simulink model "modelo"  (R2020b)
settings: Solver=ode45  StartTime=0.0  StopTime=10  MaxStep=0.005  RelTol=0.5e-3  EnableMultiTasking=on
undefined symbols (not defined in the file): B, Jt, Ke, Kt, L, Ra
settings Model: Creator=Administrador  LastModifiedBy=andre
settings DataIOCC: LimitDataPoints=on  SaveFormat=Array  SignalLoggingSaveFormat=ModelDataLogs  ReturnWorkspaceOutputs=off
settings OptimizationCC: ExpressionDepthLimit=2147483647  InitFltsAndDblsToZero=on  LifeSpan=inf
settings DebuggingCC: UnderspecifiedInitializationDetection=Classic  MergeDetectMultiDrivingBlocksExec=none  SolverPrmCheckMsg=warning  FcnCallInpInsideContextMsg=warning  StateNameClashWarn=warning  SFUnexpectedBacktrackingDiag=warning  SFNoUnconditionalDefaultTransitionDiag=warning  SFExecutionAtInitializationDiag=none  ArithmeticOperatorsInVariantConditions=warning
settings HardwareCC: ProdBitPerPointer=32  ProdBitPerSizeT=32  ProdBitPerPtrDiffT=32  ProdLargestAtomicFloat=None  ProdIntDivRoundTo=Undefined  ProdEndianess=Unspecified  ProdWordSize=32  ProdHWDeviceType=32-bit Generic
settings ModelReferenceCC: PropagateSignalLabelsOutOfModel=off
settings SFSimCC: SimUseLocalCustomCode=off  CustomCodeUndefinedFunction=UseInterfaceOnly
settings RTWCC: RTWUseLocalCustomCode=off
settings CodeAppCC: StateflowObjectComments=on
settings GRTTargetCC: TargetLangStandard=C89/C90 (ANSI)  CombineOutputUpdateFcns=off  GRTInterface=on
settings ConfigComp: CovMetricSettings=dw  CovSaveCumulativeToWorkspaceVar=on  CovSaveSingleToWorkspaceVar=on  CovExternalEMLEnable=off

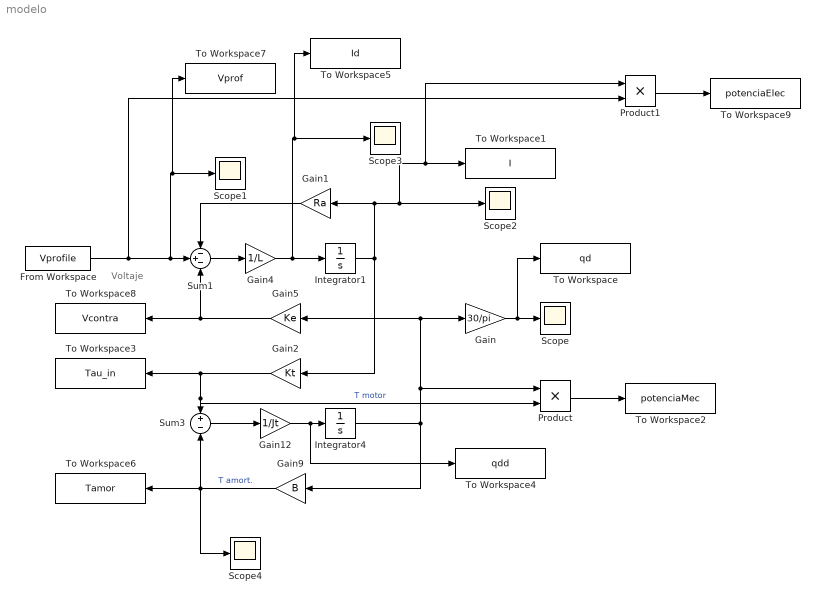
== system modelo ==
  note: Voltaje
  From Workspace : FromWorkspace  VariableName=Vprofile
  Gain : Gain  Gain=30/pi
  Gain1 : Gain  Gain=Ra
  Gain12 : Gain  Gain=1/Jt
  Gain2 : Gain  Gain=Kt
  Gain4 : Gain  Gain=1/L
  Gain5 : Gain  Gain=Ke
  Gain9 : Gain  Gain=B
  Integrator1 : Integrator
  Integrator4 : Integrator
  Product : Product
  Product1 : Product
  Scope{,1..4} (5 alike) : Scope
  Sum1 : Sum  Inputs=-+-
  Sum3 : Sum  Inputs=+-
  To Workspace : ToWorkspace  VariableName=qd  SaveFormat=Timeseries  SampleTime=-1
  To Workspace1 : ToWorkspace  VariableName=I  SaveFormat=Timeseries  SampleTime=-1
  To Workspace2 : ToWorkspace  VariableName=potenciaMec  SaveFormat=Timeseries  SampleTime=-1
  To Workspace3 : ToWorkspace  VariableName=Tau_in  SaveFormat=Timeseries  SampleTime=-1
  To Workspace4 : ToWorkspace  VariableName=qdd  SaveFormat=Timeseries  SampleTime=-1
  To Workspace5 : ToWorkspace  VariableName=Id  SaveFormat=Timeseries  SampleTime=-1
  To Workspace6 : ToWorkspace  VariableName=Tamor  SaveFormat=Timeseries  SampleTime=-1
  To Workspace7 : ToWorkspace  VariableName=Vprof  SaveFormat=Timeseries  SampleTime=-1
  To Workspace8 : ToWorkspace  VariableName=Vcontra  SaveFormat=Timeseries  SampleTime=-1
  To Workspace9 : ToWorkspace  VariableName=potenciaElec  SaveFormat=Timeseries  SampleTime=-1
  wires:
  Gain9/1 -> To Workspace6/1, Scope4/1, Sum3/2  "T amort."
  Gain12/1 -> To Workspace4/1, Integrator4/1
  Gain4/1 -> To Workspace5/1, Scope3/1, Integrator1/1
  Sum1/1 -> Gain4/1
  Sum3/1 -> Gain12/1
  Gain5/1 -> To Workspace8/1, Sum1/3
  Integrator4/1 -> Gain9/1, Product/1, Gain/1, Gain5/1
  Gain2/1 -> To Workspace3/1, Product/2, Sum3/1  "T motor"
  Gain1/1 -> Sum1/1
  Gain/1 -> To Workspace/1, Scope/1
  Product/1 -> To Workspace2/1
  Integrator1/1 -> Gain2/1, Product1/1, To Workspace1/1, Scope2/1, Gain1/1
  Product1/1 -> To Workspace9/1
  From Workspace/1 -> Product1/2, To Workspace7/1, Scope1/1, Sum1/2
